simulink model "Lateral_control_of_HST"  (R2023b)
settings: Solver=ode45  StartTime=0.0  StopTime=100  FixedStep=0.001  RelTol=1e-3
InitFcn:
  | Parameters_and_initial_conditions;
values from neighbouring files (symbols this model uses):
  A_a = 2.119e-7    (= 2.119e-07)    [Parameters_and_initial_conditions.m]
  A_v = 4.032e-7    (= 4.032e-07)    [Parameters_and_initial_conditions.m]
  b = 0.7465    [Parameters_and_initial_conditions.m]
  c_px = 0    [Parameters_and_initial_conditions.m]
  c_py = 0    [Parameters_and_initial_conditions.m]
  c_pz = 1.5e4    (= 15000)    [Parameters_and_initial_conditions.m]
  c_sx = 0    [Parameters_and_initial_conditions.m]
  c_sy = 2e4    (= 20000)    [Parameters_and_initial_conditions.m]
  c_sz = 8e4    (= 80000)    [Parameters_and_initial_conditions.m]
  d_p = 1    [Parameters_and_initial_conditions.m]
  d_s = 1    [Parameters_and_initial_conditions.m]
  f_11 = 1.12e7    (= 11200000)    [Parameters_and_initial_conditions.m]
  f_22 = 9.98e6    (= 9980000)    [Parameters_and_initial_conditions.m]
  h_cs = 0.98    [Parameters_and_initial_conditions.m]
  h_ts = 0.0945    [Parameters_and_initial_conditions.m]
  h_tw = 0.1745    [Parameters_and_initial_conditions.m]
  J_cx = 89396    [Parameters_and_initial_conditions.m]
  J_cz = 2485756    [Parameters_and_initial_conditions.m]
  J_tx = 2650    [Parameters_and_initial_conditions.m]
  J_tz = 3000    [Parameters_and_initial_conditions.m]
  J_wz = 1200    [Parameters_and_initial_conditions.m]
  k11 = 1.88e7    (= 18800000)    [Parameters_and_initial_conditions.m]
  k12 = 5.807e5    (= 580700)    [Parameters_and_initial_conditions.m]
  k13 = 3.68e6    (= 3680000)    [Parameters_and_initial_conditions.m]
  k14 = 2.64e1    (= 26.4)    [Parameters_and_initial_conditions.m]
  k21 = 1.88e7    (= 18800000)    [Parameters_and_initial_conditions.m]
  k22 = 5.807e5    (= 580700)    [Parameters_and_initial_conditions.m]
  k23 = 3.68e6    (= 3680000)    [Parameters_and_initial_conditions.m]
  k24 = 2.64e1    (= 26.4)    [Parameters_and_initial_conditions.m]
  K_gpsi = -7834    [Parameters_and_initial_conditions.m]
  K_gy = 5014    [Parameters_and_initial_conditions.m]
  k_px = 1.45e7    (= 14500000)    [Parameters_and_initial_conditions.m]
  k_py = 7.5e6    (= 7500000)    [Parameters_and_initial_conditions.m]
  k_pz = 6.65e5    (= 665000)    [Parameters_and_initial_conditions.m]
  k_sx = 2.08e5    (= 208000)    [Parameters_and_initial_conditions.m]
  k_sy = 2.08e5    (= 208000)    [Parameters_and_initial_conditions.m]
  k_sz = 3.5e5    (= 350000)    [Parameters_and_initial_conditions.m]
  kd = 1    [Parameters_and_initial_conditions.m]
  kp = 3    [Parameters_and_initial_conditions.m]
  l = 9    [Parameters_and_initial_conditions.m]
  l_t = 1.25    [Parameters_and_initial_conditions.m]
  Lambda_a = 6.125e-7    (= 6.125e-07)    [Parameters_and_initial_conditions.m]
  lambda_e = 0.05    [Parameters_and_initial_conditions.m]
  Lambda_v = 1.08e-6    (= 1.08e-06)    [Parameters_and_initial_conditions.m]
  m_c = 40000    [Parameters_and_initial_conditions.m]
  m_t = 2280    [Parameters_and_initial_conditions.m]
  m_w = 1650    [Parameters_and_initial_conditions.m]
  Omega_c = 0.8246    [Parameters_and_initial_conditions.m]
  Omega_r = 0.0206    [Parameters_and_initial_conditions.m]
  Omega_s = 0.438    [Parameters_and_initial_conditions.m]
  psi_c_dot_initial = 0    [Parameters_and_initial_conditions.m]
  psi_c_initial = 0    [Parameters_and_initial_conditions.m]
  psi_t1_dot_initial = 0    [Parameters_and_initial_conditions.m]
  psi_t1_initial = 0    [Parameters_and_initial_conditions.m]
  psi_t2_dot_initial = 0    [Parameters_and_initial_conditions.m]
  psi_t2_initial = 0    [Parameters_and_initial_conditions.m]
  psi_w1_dot_initial = 0    [Parameters_and_initial_conditions.m]
  psi_w1_initial = 0    [Parameters_and_initial_conditions.m]
  psi_w2_dot_initial = 0    [Parameters_and_initial_conditions.m]
  psi_w2_initial = 0    [Parameters_and_initial_conditions.m]
  psi_w3_dot_initial = 0    [Parameters_and_initial_conditions.m]
  psi_w3_initial = 0    [Parameters_and_initial_conditions.m]
  psi_w4_dot_initial = 0    [Parameters_and_initial_conditions.m]
  psi_w4_initial = 0    [Parameters_and_initial_conditions.m]
  r_0 = 0.4575    [Parameters_and_initial_conditions.m]
  sigma = 0.05    [Parameters_and_initial_conditions.m]
  T1 = 0.15    [Parameters_and_initial_conditions.m]
  T2 = 0.04    [Parameters_and_initial_conditions.m]
  Tff = 0.1*tau    (= 0.3)    [Parameters_and_initial_conditions.m]
  Tff2 = 0.2*tau    (= 0.6)    [Parameters_and_initial_conditions.m]
  theta_c_dot_initial = 0    [Parameters_and_initial_conditions.m]
  theta_c_initial = 0    [Parameters_and_initial_conditions.m]
  theta_t1_dot_initial = 0    [Parameters_and_initial_conditions.m]
  theta_t1_initial = 0    [Parameters_and_initial_conditions.m]
  theta_t2_dot_initial = 0    [Parameters_and_initial_conditions.m]
  theta_t2_initial = 0    [Parameters_and_initial_conditions.m]
  Tnn = 0.5*tau    (= 1.5)    [Parameters_and_initial_conditions.m]
  Tnn2 = 1*tau    (= 3)    [Parameters_and_initial_conditions.m]
  V = 75    [Parameters_and_initial_conditions.m]
  y_c_dot_initial = 0    [Parameters_and_initial_conditions.m]
  y_c_initial = 0    [Parameters_and_initial_conditions.m]
  y_t1_dot_initial = 0    [Parameters_and_initial_conditions.m]
  y_t1_initial = 0    [Parameters_and_initial_conditions.m]
  y_t2_dot_initial = 0    [Parameters_and_initial_conditions.m]
  y_t2_initial = 0    [Parameters_and_initial_conditions.m]
  y_w1_dot_initial = 0    [Parameters_and_initial_conditions.m]
  y_w1_initial = 0    [Parameters_and_initial_conditions.m]
  y_w2_dot_initial = 0    [Parameters_and_initial_conditions.m]
  y_w2_initial = 0    [Parameters_and_initial_conditions.m]
  y_w3_dot_initial = 0    [Parameters_and_initial_conditions.m]
  y_w3_initial = 0    [Parameters_and_initial_conditions.m]
  y_w4_dot_initial = 0    [Parameters_and_initial_conditions.m]
  y_w4_initial = 0    [Parameters_and_initial_conditions.m]
libraries: simulink x6, dspsrcs4 x1
(part 1 of 2)
settings Model: Creator=Sky  LastModifiedBy=19534
settings SolverCC: AlgebraicLoopSolver=TrustRegion
settings DataIOCC: ReturnWorkspaceOutputs=off
settings DebuggingCC: UnconnectedInputMsg=warning  UnconnectedOutputMsg=warning  UnconnectedLineMsg=warning  ArithmeticOperatorsInVariantConditions=warning
settings ModelReferenceCC: EnableRefExpFcnMdlSchedulingChecks=on
settings SFSimCC: CustomCodeUndefinedFunction=UseInterfaceOnly

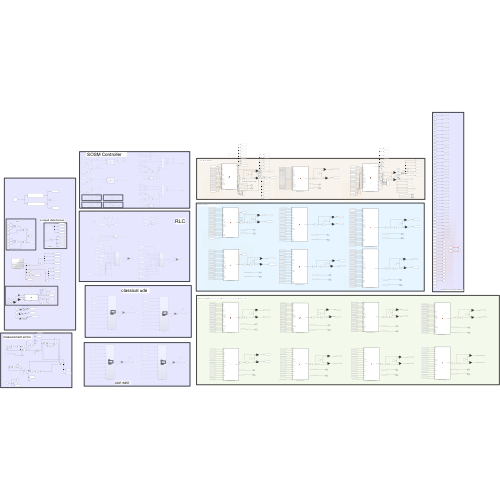
[thumbnail: Simulink's stored preview of the top-level diagram]
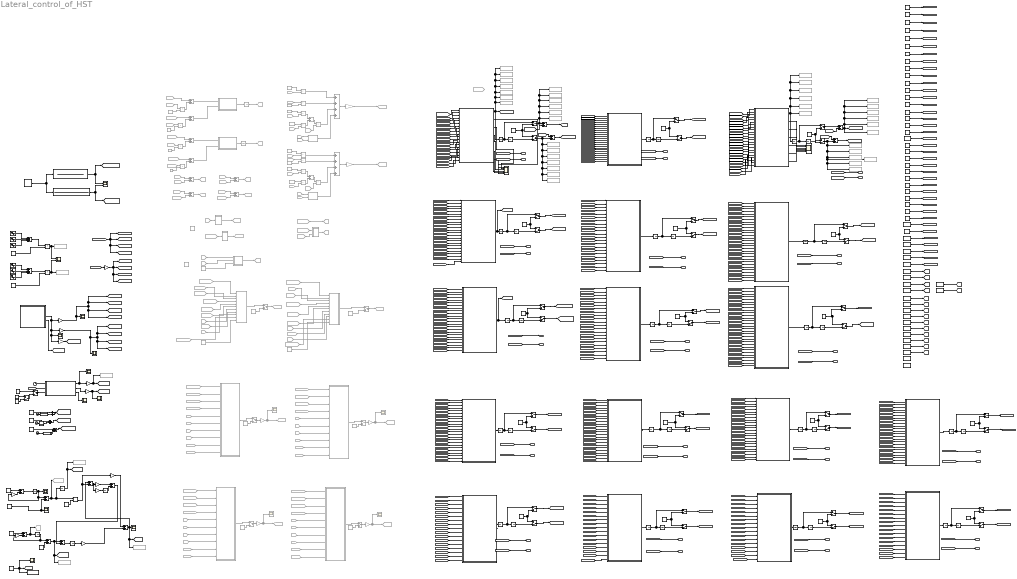
== system Lateral_control_of_HST ==
  note: classical ude
  note: 周期
  note: 非周期
  note: RLC
  note: 积分器的初值由外部m文件配置
  note: Car Body Dynamics
  note: Bogie Dynamics ( i = 1 , 2 )
  note: Wheelset Dynamics ( i = 1 , 2 , while j = 1 ; i = 3 , 4 , while j = 2 ) :
  note: Lumped disturbances
  note: measurement errors
  note: 这边是外部m文件中的系统参数导入simulink环境
  note: SOSM Controller
  note: X
  note: X_dot
  note: X_dot
  note: X
  note: UDE+MEE
  " " : Constant  Value=Lambda_v
  (3) : Sin  Amplitude=1/3  Frequency=2*pi  Phase=pi/2  SampleTime=0
  (35) : Sin  Amplitude=1/35  Frequency=6*pi  Phase=pi/2  SampleTime=0
  {0..1,23..26} (6 alike) : Constant  Commented=on  Value=0
  15 : Sin  Amplitude=1/15  Frequency=4*pi  Phase=pi/2  SampleTime=0
  3 : Sin  Amplitude=1/3  Frequency=2*pi  Phase=pi/2  SampleTime=0
  35 : Sin  Amplitude=1/35  Frequency=6*pi  Phase=pi/2  SampleTime=0
  4A_ap/pi : Constant  Value=4*0.01/pi
  4A_vp/b*pi : Constant  Value=4*0.01/(pi*0.7465)
  99 : Sin  Amplitude=1/99  Frequency=10*pi  Phase=pi/2  SampleTime=0
  Add : Sum  Inputs=+-+
  Add1 : Sum  Inputs=+++
  Add{9..10,14..21,24..25,49} (13 alike) : Sum
  Add{8,38..40,44,48} (6 alike) : Sum  Commented=on
  Add{41..42,45..46} (4 alike) : Sum  Commented=on  Inputs=+-
  Add43 : Sum  Commented=on  Inputs=++++
  Add47 : Sum  Commented=on  Inputs=++++
  Atan2 : Trigonometry  Operator=atan2
  Band-Limited White Noise : simulink/Sources/Band-Limited White Noise  Cov=[0.1]  Ts=0.001  seed=[100]
  Band-Limited White Noise1 : simulink/Sources/Band-Limited White Noise  Cov=[1e-12]  Ts=0.001  seed=[1001]
  Band-Limited White Noise4 : simulink/Sources/Band-Limited White Noise  Cov=[0.000000000418]  Ts=0.01  seed=[23341]
  Band-Limited White Noise5 : simulink/Sources/Band-Limited White Noise  Cov=[0.00000045]  Ts=0.01  seed=[23341]
  Band-Limited White Noise6 : simulink/Sources/Band-Limited White Noise  Cov=[0.00000000006985]  Ts=0.01  seed=[23341]
  Band-Limited White Noise7 : simulink/Sources/Band-Limited White Noise  Cov=[0.00000000487]  Ts=0.01  seed=[23341]
  Clock{2,9..10,17} (4 alike) : Clock
  Constant{1..17} (17 alike) : Constant  Value=0
  Constant19 : Constant  Commented=on  Value=0.25
  Constant21 : Constant  Commented=on  Value=0.25
  Constant{23,40,44..45,56..57} (6 alike) : Constant  Commented=on  Value=50
  Constant30 : Constant  Value=T1
  Constant33 : Constant  Value=T2
  Constant34 : Constant  Value=9.8
  Constant41 : Constant  Commented=on  Value=15
  Constant42 : Constant  Value=A_a
  Constant43 : Constant  Value=A_v
  Differential equation of psi_c : MATLAB Function  TreatAsAtomicUnit=on
  Differential equation of psi_t1 : MATLAB Function  TreatAsAtomicUnit=on
  Differential equation of psi_t2 : MATLAB Function  TreatAsAtomicUnit=on
  "Differential equation of psi_w1 " : MATLAB Function  TreatAsAtomicUnit=on
  Differential equation of psi_w2 : MATLAB Function  TreatAsAtomicUnit=on
  Differential equation of psi_w3 : MATLAB Function  TreatAsAtomicUnit=on
  Differential equation of psi_w4 : MATLAB Function  TreatAsAtomicUnit=on
  Differential equation of theta_c : MATLAB Function  TreatAsAtomicUnit=on
  Differential equation of theta_t1 : MATLAB Function  TreatAsAtomicUnit=on
  Differential equation of theta_t2 : MATLAB Function  TreatAsAtomicUnit=on
  Differential equation of y_c : MATLAB Function  TreatAsAtomicUnit=on
  Differential equation of y_t1 : MATLAB Function  TreatAsAtomicUnit=on
  Differential equation of y_t2 : MATLAB Function  TreatAsAtomicUnit=on
  Differential equation of y_w1 : MATLAB Function  TreatAsAtomicUnit=on
  Differential equation of y_w2 : MATLAB Function  TreatAsAtomicUnit=on
  Differential equation of y_w3 : MATLAB Function  TreatAsAtomicUnit=on
  Differential equation of y_w4 : MATLAB Function  TreatAsAtomicUnit=on
  F_wind : MATLAB Function  TreatAsAtomicUnit=on
  From1069 : From  Commented=on  GotoTag=noise_ddx
  From415 : From  Commented=on  GotoTag=K_sy
  From416 : From  Commented=on  GotoTag=C_sy
  From417 : From  Commented=on  GotoTag=M_c
  From418 : From  Commented=on  GotoTag=K_sy
  From419 : From  Commented=on  GotoTag=C_sy
  From420 : From  Commented=on  GotoTag=M_c
  From{423,812,817,822} (4 alike) : From  Commented=on  GotoTag=y_t1_dot
  From425 : From  Commented=on  GotoTag=y_t1
  From{426,428,435,803,819,829,854,861,881,884} (10 alike) : From  Commented=on  GotoTag=y_c
  From{427,430,436..437,813,815,821,831,855,863,882,886} (12 alike) : From  Commented=on  GotoTag=y_c_dot
  From429 : From  Commented=on  GotoTag=d_hat
  From431 : From  Commented=on  GotoTag=y_t2_dot
  From432 : From  Commented=on  GotoTag=y_t2
  From449 : From  Commented=on  GotoTag=d_hat
  From455 : From  Commented=on  GotoTag=z_1
  From457 : From  Commented=on  GotoTag=alpha_1_dot
  From466 : From  Commented=on  GotoTag=z_1
  From472 : From  Commented=on  GotoTag=alpha_1
  From474 : From  Commented=on  GotoTag=d_hat
  From475 : From  Commented=on  GotoTag=alpha_1_dot
  From476 : From  Commented=on  GotoTag=z_1
  From480 : From  Commented=on  GotoTag=z_2
  From804 : From  Commented=on  GotoTag=y_t1
  From814 : From  Commented=on  GotoTag=y_c_ddot
  From816 : From  Commented=on  GotoTag=y_t1_ddot
  From{818,828,833,839} (4 alike) : From  Commented=on  GotoTag=ic
  From820 : From  Commented=on  GotoTag=y_t1
  From823 : From  Commented=on  GotoTag=Xc1_dot
  From824 : From  Commented=on  GotoTag=Xc1
  From825 : From  Commented=on  GotoTag=Xc1_dot
  From826 : From  Commented=on  GotoTag=Xc1
  From827 : From  Commented=on  GotoTag=Xc1
  From830 : From  Commented=on  GotoTag=y_t2
  From832 : From  Commented=on  GotoTag=y_t2_dot
  From834 : From  Commented=on  GotoTag=Xc2_dot
  From835 : From  Commented=on  GotoTag=Xc2
  From836 : From  Commented=on  GotoTag=Xc2_dot
  From837 : From  Commented=on  GotoTag=Xc2
  From838 : From  Commented=on  GotoTag=Xc2
  From{856,869,883,890} (4 alike) : From  Commented=on  GotoTag=theta_c
  From{862,870,885,891} (4 alike) : From  Commented=on  GotoTag=theta_c_dot
  From864 : From  Commented=on  GotoTag=k21
  From865 : From  Commented=on  GotoTag=k22
  From868 : From  Commented=on  GotoTag=k23
  From871 : From  Commented=on  GotoTag=k24
  From{872,878,893,899} (4 alike) : From  Commented=on  GotoTag=f_1
  From{873,879,894,900} (4 alike) : From  Commented=on  GotoTag=f_2
  From874 : From  Commented=on  GotoTag=k11
  From875 : From  Commented=on  GotoTag=k12
  From876 : From  Commented=on  GotoTag=k13
  From877 : From  Commented=on  GotoTag=k14
  From887 : From  Commented=on  GotoTag=k11
  From888 : From  Commented=on  GotoTag=k12
  From889 : From  Commented=on  GotoTag=k13
  From892 : From  Commented=on  GotoTag=k14
  From895 : From  Commented=on  GotoTag=k11
  From896 : From  Commented=on  GotoTag=k12
  From897 : From  Commented=on  GotoTag=k13
  From898 : From  Commented=on  GotoTag=k14
  Gain{,3..4,6,10,21} (6 alike) : Gain
  Gain1 : Gain  Gain=5
  Gain2 : Gain  Gain=0.04
  Gain23 : Gain  Commented=on  Gain=16.7
  Gain24 : Gain  Commented=on  Gain=16.7
  Gain{26..29} (4 alike) : Gain  Commented=on
  Gain5 : Gain  Gain=0
  Gain7 : Gain  Gain=-0.01315789
  Gain8 : Gain  Gain=-0.05263158
  Gain9 : Gain  Gain=0.001
  Goto154 : Goto  Commented=on  GotoTag=noise_ddx
  Goto155 : Goto  Commented=on  GotoTag=noise_ddphi
  Goto162 : Goto  Commented=on  GotoTag=ic
  Goto163 : Goto  Commented=on  GotoTag=it
  Goto164 : Goto  Commented=on  GotoTag=Xc1
  Goto165 : Goto  Commented=on  GotoTag=Xc1_dot
  Goto{45,166,176,181} (4 alike) : Goto  Commented=on  GotoTag=f_1
  Goto167 : Goto  Commented=on  GotoTag=Xc2
  Goto168 : Goto  Commented=on  GotoTag=Xc2_dot
  Goto17 : Goto  Commented=on  GotoTag=z_1
  Goto{48,173,179,182} (4 alike) : Goto  Commented=on  GotoTag=f_2
  Goto20 : Goto  Commented=on  GotoTag=d_hat
  Goto39 : Goto  Commented=on  GotoTag=alpha_1
  Goto42 : Goto  Commented=on  GotoTag=alpha_1_dot
  Goto51 : Goto  Commented=on  GotoTag=z_2
  Integrator : Integrator  InitialCondition=y_c_dot_initial
  Integrator1 : Integrator  InitialCondition=y_c_initial
  Integrator10 : Integrator  InitialCondition=psi_t1_dot_initial
  Integrator11 : Integrator  InitialCondition=psi_t1_initial
  Integrator12 : Integrator  InitialCondition=psi_t2_initial
  Integrator13 : Integrator  InitialCondition=psi_t2_dot_initial
  Integrator14 : Integrator  InitialCondition=theta_t1_dot_initial
  Integrator15 : Integrator  InitialCondition=theta_t1_initial
  Integrator16 : Integrator  InitialCondition=theta_t2_dot_initial
  Integrator17 : Integrator  InitialCondition=theta_t2_initial
  Integrator18 : Integrator  InitialCondition=y_w1_dot_initial
  Integrator19 : Integrator  InitialCondition=y_w1_initial
  Integrator2 : Integrator  InitialCondition=psi_c_dot_initial
  Integrator20 : Integrator  InitialCondition=y_w2_dot_initial
  Integrator21 : Integrator  InitialCondition=y_w2_initial
  Integrator22 : Integrator  InitialCondition=y_w3_dot_initial
  Integrator23 : Integrator  InitialCondition=y_w3_initial
  Integrator24 : Integrator  InitialCondition=y_w4_initial
  Integrator25 : Integrator  InitialCondition=y_w4_dot_initial
  Integrator26 : Integrator  InitialCondition=psi_w1_dot_initial
  Integrator27 : Integrator  InitialCondition=psi_w1_initial
  Integrator28 : Integrator  InitialCondition=psi_w2_dot_initial
  Integrator29 : Integrator  InitialCondition=psi_w2_initial
  Integrator3 : Integrator  InitialCondition=psi_c_initial
  Integrator30 : Integrator  InitialCondition=psi_w3_dot_initial
  Integrator31 : Integrator  InitialCondition=psi_w3_initial
  Integrator32 : Integrator  InitialCondition=psi_w4_dot_initial
  Integrator33 : Integrator  InitialCondition=psi_w4_initial
  Integrator{34..38} (5 alike) : Integrator
  Integrator4 : Integrator  InitialCondition=theta_c_dot_initial
  Integrator41 : Integrator  Commented=on  LimitOutput=on  UpperSaturationLimit=80  LowerSaturationLimit=0
  Integrator42 : Integrator  Commented=on
  Integrator5 : Integrator  InitialCondition=theta_c_initial
  Integrator6 : Integrator  InitialCondition=y_t1_dot_initial
  Integrator7 : Integrator  InitialCondition=y_t1_initial
  Integrator8 : Integrator  InitialCondition=y_t2_dot_initial
  Integrator9 : Integrator  InitialCondition=y_t2_initial
  J_cx : Constant  Value=J_cx
  J_cz : Constant  Value=J_cz
  "J_tx " : Constant  Value=J_tx
  "J_tz " : Constant  Value=J_tz
  J_wz : Constant  Value=J_wz
  K_gpsi : Constant  Value=K_gpsi
  K_gy : Constant  Value=K_gy
  Lambda_a : Constant  Value=Lambda_a
  MATLAB Function10 : MATLAB Function  Commented=on  TreatAsAtomicUnit=on
  MATLAB Function16 : MATLAB Function  TreatAsAtomicUnit=on
  MATLAB Function5 : MATLAB Function  Commented=on  TreatAsAtomicUnit=on
  MATLAB Function6 : MATLAB Function  Commented=on  TreatAsAtomicUnit=on
  MATLAB Function7 : MATLAB Function  Commented=on  TreatAsAtomicUnit=on
  MATLAB Function8 : MATLAB Function  TreatAsAtomicUnit=on
  MATLAB Function9 : MATLAB Function  TreatAsAtomicUnit=on
  M_t : Constant  Value=m_t
  M_w : Constant  Value=m_w
  Manual Switch{,35,56..59} (6 alike) : ManualSwitch  Commented=on
  Manual Switch{1..2,4,6,8,10,12,14,16,18,20,22,24,26,28,30,32,54} (18 alike) : ManualSwitch
  Manual Switch{3,5,7,9,11,13,15,17,19,21,23,25,27,29,31,33..34,53} (18 alike) : ManualSwitch  CurrentSetting=0
  Omega_c : Constant  Value=Omega_c
  Omega_r : Constant  Value=Omega_r
  Omega_s : Constant  Value=Omega_s
  Product1 : Product
  Product24 : Product
  Product{46..59} (14 alike) : Product  Commented=on
  Scope : Scope  NumInputPorts=2
  Scope1 : Scope  NumInputPorts=2
  Scope{10,14,33..34} (4 alike) : Scope  Commented=on
  Scope{2..4,7..8,25,30..32,35} (10 alike) : Scope
  Scope40 : Scope  NumInputPorts=6
  Scope49 : Scope  NumInputPorts=6
  Subsystem10 : Subsystem  Commented=on
  Subsystem11 : Subsystem  Commented=on
  Subsystem3 : Subsystem  Commented=on
  Subsystem7 : Subsystem  Commented=on
  Subsystem8 : Subsystem  Commented=on
  Subsystem9 : Subsystem  Commented=on
  Subtract : Sum  Inputs=+-
  Subtract1 : Sum  Inputs=+-
  Tff : Constant  Value=Tff
  Tff2 : Constant  Value=Tff2
  Tnn : Constant  Value=Tnn
  Tnn2 : Constant  Value=Tnn2
  To Workspace1 : ToWorkspace  Commented=on  VariableName=wind_20  SaveFormat=Timeseries  SampleTime=-1
  To Workspace10 : ToWorkspace  Commented=on  VariableName=v_passive_n  SaveFormat=Timeseries  SampleTime=-1
  To Workspace11 : ToWorkspace  Commented=on  VariableName=acc_passive_n  SaveFormat=Timeseries  SampleTime=-1
  To Workspace12 : ToWorkspace  Commented=on  VariableName=acc_sosm_n  SaveFormat=Timeseries  SampleTime=-1
  To Workspace13 : ToWorkspace  Commented=on  VariableName=acc_rlc_n  SaveFormat=Timeseries  SampleTime=-1
  To Workspace14 : ToWorkspace  Commented=on  VariableName=acc_ude_n  SaveFormat=Timeseries  SampleTime=-1
  To Workspace15 : ToWorkspace  Commented=on  VariableName=pacc_sosm_n  SaveFormat=Timeseries  SampleTime=-1
  To Workspace16 : ToWorkspace  Commented=on  VariableName=acc_mee  SaveFormat=Timeseries  SampleTime=-1
  To Workspace17 : ToWorkspace  Commented=on  VariableName=v_sosm_n  SaveFormat=Timeseries  SampleTime=-1
  To Workspace18 : ToWorkspace  Commented=on  VariableName=theta_cl  SaveFormat=Timeseries  SampleTime=-1
  To Workspace19 : ToWorkspace  Commented=on  VariableName=noise_v  SaveFormat=Timeseries  SampleTime=-1
  To Workspace2 : ToWorkspace  Commented=on  VariableName=phic_v_sosm_n  SaveFormat=Timeseries  SampleTime=-1
  To Workspace20 : ToWorkspace  Commented=on  VariableName=noise_w  SaveFormat=Timeseries  SampleTime=-1
  To Workspace21 : ToWorkspace  Commented=on  VariableName=v_rlc_n  SaveFormat=Timeseries  SampleTime=-1
  To Workspace22 : ToWorkspace  Commented=on  VariableName=v_ude_n  SaveFormat=Timeseries  SampleTime=-1
  To Workspace23 : ToWorkspace  Commented=on  VariableName=v_mee  SaveFormat=Timeseries  SampleTime=-1
  To Workspace24 : ToWorkspace  Commented=on  VariableName=phic_sosm_n  SaveFormat=Timeseries  SampleTime=-1
  To Workspace25 : ToWorkspace  Commented=on  VariableName=phic_rlc_n  SaveFormat=Timeseries  SampleTime=-1
  To Workspace26 : ToWorkspace  Commented=on  VariableName=phic_ude_n  SaveFormat=Timeseries  SampleTime=-1
  To Workspace27 : ToWorkspace  Commented=on  VariableName=phic_mee  SaveFormat=Timeseries  SampleTime=-1
  To Workspace28 : ToWorkspace  Commented=on  VariableName=phic_v_rlc_n  SaveFormat=Timeseries  SampleTime=-1
  To Workspace29 : ToWorkspace  Commented=on  VariableName=phic_v_ude_n  SaveFormat=Timeseries  SampleTime=-1
  To Workspace3 : ToWorkspace  Commented=on  VariableName=ya  SaveFormat=Timeseries  SampleTime=-1
  To Workspace30 : ToWorkspace  Commented=on  VariableName=phic_v_mee  SaveFormat=Timeseries  SampleTime=-1
  To Workspace31 : ToWorkspace  Commented=on  VariableName=phic_v_passive_n  SaveFormat=Timeseries  SampleTime=-1
  To Workspace32 : ToWorkspace  Commented=on  VariableName=pacc_rlc_n  SaveFormat=Timeseries  SampleTime=-1
  To Workspace33 : ToWorkspace  Commented=on  VariableName=pacc_ude_n  SaveFormat=Timeseries  SampleTime=-1
  To Workspace34 : ToWorkspace  Commented=on  VariableName=pacc_mee  SaveFormat=Timeseries  SampleTime=-1
  To Workspace35 : ToWorkspace  Commented=on  VariableName=pacc_passive_n  SaveFormat=Timeseries  SampleTime=-1
  To Workspace36 : ToWorkspace  Commented=on  VariableName=acc_tau_5  SaveFormat=Timeseries  SampleTime=-1
  To Workspace37 : ToWorkspace  Commented=on  VariableName=yc_tau_10  SaveFormat=Timeseries  SampleTime=-1
  To Workspace38 : ToWorkspace  Commented=on  VariableName=acc_mee_n  SaveFormat=Timeseries  SampleTime=-1
  To Workspace39 : ToWorkspace  Commented=on  VariableName=yc_mee_n  SaveFormat=Timeseries  SampleTime=-1
  To Workspace4 : ToWorkspace  Commented=on  VariableName=yc_passive_n  SaveFormat=Timeseries  SampleTime=-1
  To Workspace40 : ToWorkspace  Commented=on  VariableName=pacc_mee_n  SaveFormat=Timeseries  SampleTime=-1
  To Workspace41 : ToWorkspace  Commented=on  VariableName=phic_mee_n  SaveFormat=Timeseries  SampleTime=-1
  To Workspace42 : ToWorkspace  Commented=on  VariableName=phic_v_mee_n  SaveFormat=Timeseries  SampleTime=-1
  To Workspace43 : ToWorkspace  Commented=on  VariableName=v_mee_n  SaveFormat=Timeseries  SampleTime=-1
  To Workspace44 : ToWorkspace  Commented=on  VariableName=noise_theata  SaveFormat=Timeseries  SampleTime=-1
  To Workspace46 : ToWorkspace  VariableName=yczaosheng  SaveFormat=Timeseries  SampleTime=-1
  To Workspace5 : ToWorkspace  Commented=on  VariableName=phic_passive_n  SaveFormat=Timeseries  SampleTime=-1
  To Workspace6 : ToWorkspace  Commented=on  VariableName=yc_sosm_n  SaveFormat=Timeseries  SampleTime=-1
  To Workspace7 : ToWorkspace  Commented=on  VariableName=yc_rlc_n  SaveFormat=Timeseries  SampleTime=-1
  To Workspace8 : ToWorkspace  Commented=on  VariableName=yc_ude_n  SaveFormat=Timeseries  SampleTime=-1
  To Workspace9 : ToWorkspace  Commented=on  VariableName=yc_mee  SaveFormat=Timeseries  SampleTime=-1
  Transfer Fcn2 : TransferFcn  Numerator=[sqrt(2*pi*A_a*V^3*Omega_c^2)]  Denominator=conv([1 V*Omega_r], [1 V*Omega_c])
  Transfer Fcn3 : TransferFcn  Numerator=[sqrt(2*pi*A_v*b^-2*V^3*Omega_c^2) 0]  Denominator=conv(conv([1 V*Omega_r], [1 V*Omega_c]), [1 V*Omega_s])
  UDE+MEE4（新）10 : Subsystem  Commented=on
  UDE+MEE4（新）8 : Subsystem  Commented=on
  UDE1 : Subsystem  Commented=on
  UDE2 : Subsystem  Commented=on
  V : Constant  Value=V
  b : Constant  Value=b
  c4 : Constant  Commented=on  Value=1232*6
  c5 : Constant  Commented=on  Value=1929*6
  c6 : Constant  Commented=on  Value=1232*6
  c7 : Constant  Commented=on  Value=1929*6
  c_px : Constant  Value=c_px
  c_py : Constant  Value=c_py
  "c_pz " : Constant  Value=c_pz
  c_sx : Constant  Value=c_sx
  "c_sy " : Constant  Value=c_sy
  "c_sz " : Constant  Value=c_sz
  d_p : Constant  Value=d_p
  d_s : Constant  Value=d_s
  disturbance and noise : Subsystem
  f_11 : Constant  Value=f_11
  f_22 : Constant  Value=f_22
  h_cs : Constant  Value=h_cs
  "h_ts " : Constant  Value=h_ts
  h_tw : Constant  Value=h_tw
  k1 : Constant  Value=k21
  k1'2 : Constant  Commented=on  Value=1929*6
  k1'3 : Constant  Commented=on  Value=1929*6
  k11 : Constant  Value=k11
  k12 : Constant  Value=k12
  k13 : Constant  Value=k13
  k14 : Constant  Value=k14
  k2 : Constant  Value=k22
  k23 : Constant  Value=k23
  k24 : Constant  Value=k24
  k4 : Constant  Commented=on  Value=5100*6
  k5 : Constant  Commented=on  Value=5100*6
  k_px : Constant  Value=k_px
  "k_py " : Constant  Value=k_py
  k_pz : Constant  Value=k_pz
  k_sx : Constant  Value=k_sx
  k_sy : Constant  Value=k_sy
  k_sz : Constant  Value=k_sz
  kd : Constant  Value=kd
  kp : Constant  Value=kp
  l_c : Constant  Value=l
  l_t : Constant  Value=l_t
  lambda_e : Constant  Value=lambda_e
  m_c : Constant  Value=m_c
  r_0 : Constant  Value=r_0
  sigma : Constant  Value=sigma
  w_wind : Constant  Value=0
  w_wind1 : Constant  Value=10
  w_wind4 : Constant  Value=20
  y_c : Outport  VectorParamsAs1DForOutWhenUnconnected=off
  y_c_dot : Outport  Port=2  VectorParamsAs1DForOutWhenUnconnected=off
  psi_c : Outport  Port=3  VectorParamsAs1DForOutWhenUnconnected=off
  psi_c_dot : Outport  Port=4  VectorParamsAs1DForOutWhenUnconnected=off
  theta_c : Outport  Port=5  VectorParamsAs1DForOutWhenUnconnected=off
  theta_c_dot : Outport  Port=6  VectorParamsAs1DForOutWhenUnconnected=off
  y_t1 : Outport  Port=7  VectorParamsAs1DForOutWhenUnconnected=off
  y_t1_dot : Outport  Port=8  VectorParamsAs1DForOutWhenUnconnected=off
  y_t2 : Outport  Port=9  VectorParamsAs1DForOutWhenUnconnected=off
  y_t2_dot : Outport  Port=10  VectorParamsAs1DForOutWhenUnconnected=off
  psi_t1 : Outport  Port=11  VectorParamsAs1DForOutWhenUnconnected=off
  psi_t1_dot : Outport  Port=12  VectorParamsAs1DForOutWhenUnconnected=off
  psi_t2 : Outport  Port=13  VectorParamsAs1DForOutWhenUnconnected=off
  psi_t2_dot : Outport  Port=14  VectorParamsAs1DForOutWhenUnconnected=off
  theta_t1 : Outport  Port=15  VectorParamsAs1DForOutWhenUnconnected=off
  theta_t1_dot : Outport  Port=16  VectorParamsAs1DForOutWhenUnconnected=off
  theta_t2 : Outport  Port=17  VectorParamsAs1DForOutWhenUnconnected=off
  theta_t2_dot : Outport  Port=18  VectorParamsAs1DForOutWhenUnconnected=off
  y_w1 : Outport  Port=19  VectorParamsAs1DForOutWhenUnconnected=off
  y_w1_dot : Outport  Port=20  VectorParamsAs1DForOutWhenUnconnected=off
  y_w2 : Outport  Port=21  VectorParamsAs1DForOutWhenUnconnected=off
  y_w2_dot : Outport  Port=22  VectorParamsAs1DForOutWhenUnconnected=off
  y_w3 : Outport  Port=23  VectorParamsAs1DForOutWhenUnconnected=off
  y_w3_dot : Outport  Port=24  VectorParamsAs1DForOutWhenUnconnected=off
  y_w4 : Outport  Port=25  VectorParamsAs1DForOutWhenUnconnected=off
  y_w4_dot : Outport  Port=26  VectorParamsAs1DForOutWhenUnconnected=off
  psi_w1 : Outport  Port=27  VectorParamsAs1DForOutWhenUnconnected=off
  psi_w1_dot : Outport  Port=28  VectorParamsAs1DForOutWhenUnconnected=off
  psi_w2 : Outport  Port=29  VectorParamsAs1DForOutWhenUnconnected=off
  psi_w2_dot : Outport  Port=30  VectorParamsAs1DForOutWhenUnconnected=off
  psi_w3 : Outport  Port=31  VectorParamsAs1DForOutWhenUnconnected=off
  psi_w3_dot : Outport  Port=32  VectorParamsAs1DForOutWhenUnconnected=off
  psi_w4 : Outport  Port=33  VectorParamsAs1DForOutWhenUnconnected=off
  psi_w4_dot : Outport  Port=34  VectorParamsAs1DForOutWhenUnconnected=off
  wires:
  [y_c] -> Differential equation of y_c/3(y_c)
  [f_1] -> Differential equation of y_c/18(f_1)
  [f_2] -> Differential equation of y_c/19(f_2)
  [psi_c] -> Differential equation of psi_c/3(psi_c)
  [psi_c_dot] -> Differential equation of psi_c/4(psi_c_dot)
  [f_1] -> Differential equation of psi_c/23(f_1)
  [f_2] -> Differential equation of psi_c/24(f_2)
  [psi_c] -> psi_c/1
  [psi_c_dot] -> psi_c_dot/1
  [y_c_dot] -> y_c_dot/1
  Integrator4/1 -> Manual Switch2/1, Integrator5/1  "d_phi_real"
  [theta_c] -> Differential equation of theta_c/5(theta_c)
  [theta_c_dot] -> Differential equation of theta_c/13(theta_c_dot)
  [y_c_dot] -> Differential equation of theta_c/12(y_c_dot)
  [theta_c_dot] -> Differential equation of y_c/13(theta_c_dot)
  [theta_c] -> Differential equation of y_c/5(theta_c)
  [y_c] -> Differential equation of theta_c/3(y_c)
  [theta_c] -> theta_c/1
  [theta_c_dot] -> theta_c_dot/1
  Differential equation of y_t1/1(y_t1_ddot) -> [y_t1_ddot], Integrator6/1
  [psi_c] -> Differential equation of y_t1/5(psi_c)
  Differential equation of y_t2/1(y_t2_ddot) -> [y_t2_ddot], Integrator8/1
  [y_t2] -> y_t2/1
  [y_t2_dot] -> y_t2_dot/1
  [y_t1_dot] -> y_t1_dot/1
  [y_t1] -> y_t1/1
  Differential equation of psi_t1/1(psi_t1_ddot) -> Integrator10/1
  [psi_t1_dot] -> psi_t1_dot/1
  [psi_t1] -> psi_t1/1
  Differential equation of psi_t2/1(psi_t2_ddot) -> Integrator13/1
  [psi_t2] -> psi_t2/1
  [psi_t2_dot] -> psi_t2_dot/1
  Differential equation of theta_t1/1(theta_t1_ddot) -> Integrator14/1
  [theta_t1] -> theta_t1/1
  [theta_t1_dot] -> theta_t1_dot/1
  Differential equation of theta_t2/1(theta_t2_ddot) -> Integrator16/1
  [theta_t2] -> theta_t2/1
  [theta_t2_dot] -> theta_t2_dot/1
  Differential equation of y_w1/1(y_w1_ddot) -> Integrator18/1
  [y_w1_dot] -> y_w1_dot/1
  [y_w1] -> y_w1/1
  Differential equation of y_w2/1(y_w2_ddot) -> Integrator20/1
  [y_w2_dot] -> y_w2_dot/1
  [y_w2] -> y_w2/1
  Differential equation of y_w3/1(y_w3_ddot) -> Integrator22/1
  [y_w3_dot] -> y_w3_dot/1
  [y_w3] -> y_w3/1
  Differential equation of y_w4/1(y_w4_ddot) -> Integrator25/1
  [y_w4_dot] -> y_w4_dot/1
  [y_w4] -> y_w4/1
  "Differential equation of psi_w1 "/1(psi_w1_ddot) -> Integrator26/1
  [psi_w1_dot] -> psi_w1_dot/1
  [psi_w1] -> psi_w1/1
  Differential equation of psi_w2/1(psi_w2_ddot) -> Integrator28/1
  [psi_w2_dot] -> psi_w2_dot/1
  [psi_w2] -> psi_w2/1
  Differential equation of psi_w3/1(psi_w3_ddot) -> Integrator30/1
  [psi_w3_dot] -> psi_w3_dot/1
  [psi_w3] -> psi_w3/1
  Differential equation of psi_w4/1(psi_w4_ddot) -> Integrator32/1
  [psi_w4_dot] -> psi_w4_dot/1
  [psi_w4] -> psi_w4/1
  [M_c] -> Differential equation of y_c/1(m_c)
  [h_cs] -> Differential equation of y_c/4(h_cs)
  [y_t1] -> Differential equation of y_c/6(y_t1)
  [y_t2] -> Differential equation of y_c/7(y_t2)
  [h_ts] -> Differential equation of y_c/8(h_ts)
  [theta_t1] -> Differential equation of y_c/9(theta_t1)
  [C_sy] -> Differential equation of y_c/11(c_sy)
  [theta_t2] -> Differential equation of y_c/10(theta_t2)
  [y_t1_dot] -> Differential equation of y_c/14(y_t1_dot)
  [y_t2_dot] -> Differential equation of y_c/15(y_t2_dot)
  [theta_t2_dot] -> Differential equation of y_c/17(theta_t2_dot)
  [theta_t1_dot] -> Differential equation of y_c/16(theta_t1_dot)
  [J_cz] -> Differential equation of psi_c/1(J_cz)
  [k_sx] -> Differential equation of psi_c/2(k_sx)
  [psi_t1] -> Differential equation of psi_c/5(psi_t1)
  [psi_t2] -> Differential equation of psi_c/6(psi_t2)
  [d_s] -> Differential equation of psi_c/7(d_s)
  [c_sx] -> Differential equation of psi_c/8(c_sx)
  [psi_t1_dot] -> Differential equation of psi_c/9(psi_t1_dot)
  [psi_t2_dot] -> Differential equation of psi_c/10(psi_t2_dot)
  [K_sy] -> Differential equation of psi_c/11(k_sy)
  [l] -> Differential equation of psi_c/12(l)
  [y_t1] -> Differential equation of psi_c/13(y_t1)
  [y_t1_dot] -> Differential equation of psi_c/14(y_t1_dot)
  [y_t2] -> Differential equation of psi_c/15(y_t2)
  [y_t2_dot] -> Differential equation of psi_c/16(y_t2_dot)
  [h_ts] -> Differential equation of psi_c/17(h_ts)
  [theta_t1] -> Differential equation of psi_c/18(theta_t1)
  [theta_t1_dot] -> Differential equation of psi_c/19(theta_t1_dot)
  [theta_t2] -> Differential equation of psi_c/20(theta_t2)
  [theta_t2_dot] -> Differential equation of psi_c/21(theta_t2_dot)
  [C_sy] -> Differential equation of psi_c/22(c_sy)
  [K_sy] -> Differential equation of y_c/2(k_sy)
  [m_w] -> Differential equation of y_w1/1(m_w)
  [k_py] -> Differential equation of y_w1/2(k_py)
  [y_t1] -> Differential equation of y_w1/3(y_t1)
  [b] -> Differential equation of y_w1/4(b)
  [psi_t1] -> Differential equation of y_w1/5(psi_t1)
  [h_tp] -> Differential equation of y_w1/6(h_tp)
  [theta_t1] -> Differential equation of y_w1/7(theta_t1)
  [y_w1] -> Differential equation of y_w1/8(y_w1)
  [c_py] -> Differential equation of y_w1/9(c_py)
  [y_t1_dot] -> Differential equation of y_w1/10(y_t1_dot)
  [psi_t1_dot] -> Differential equation of y_w1/11(psi_t1_dot)
  [theta_t1_dot] -> Differential equation of y_w1/12(theta_t1_dot)
  [y_w1_dot] -> Differential equation of y_w1/13(y_w1_dot)
  [f_22] -> Differential equation of y_w1/14(f_22)
  [V] -> Differential equation of y_w1/15(V)
  [sigma] -> Differential equation of y_w1/16(sigma)
  [r_0] -> Differential equation of y_w1/17(r_0)
  [a] -> Differential equation of y_w1/18(a)
  [y_a1_dot] -> Differential equation of y_w1/19(y_a1_dot)
  [theta_cl1_dot] -> Differential equation of y_w1/20(theta_cl1_dot)
  [psi_w1] -> Differential equation of y_w1/21(psi_w1)
  [K_gy] -> Differential equation of y_w1/22(K_gy)
  [y_a1] -> Differential equation of y_w1/23(y_a1)
  [theta_cl1] -> Differential equation of y_w1/24(theta_cl1)
  [J_wz] -> "Differential equation of psi_w1 "/1(J_wz)
  [k_px] -> "Differential equation of psi_w1 "/2(k_px)
  [psi_t1] -> "Differential equation of psi_w1 "/3(psi_t1)
  [psi_w1] -> "Differential equation of psi_w1 "/4(psi_w1)
  [d_p] -> "Differential equation of psi_w1 "/5(d_p)
  [c_px] -> "Differential equation of psi_w1 "/6(c_px)
  [psi_t1_dot] -> "Differential equation of psi_w1 "/7(psi_t1_dot)
  [psi_w1_dot] -> "Differential equation of psi_w1 "/8(psi_w1_dot)
  [f_11] -> "Differential equation of psi_w1 "/9(f_11)
  [lambda_e] -> "Differential equation of psi_w1 "/10(lambda_e)
  [y_w1] -> "Differential equation of psi_w1 "/11(y_w1)
  [y_a1] -> "Differential equation of psi_w1 "/12(y_a1)
  [theta_cl1] -> "Differential equation of psi_w1 "/13(theta_cl1)
  [V] -> "Differential equation of psi_w1 "/14(V)
  [K_gpsi] -> "Differential equation of psi_w1 "/15(K_gpsi)
  [J_wz] -> Differential equation of psi_w2/1(J_wz)
  [k_px] -> Differential equation of psi_w2/2(k_px)
  [psi_t1] -> Differential equation of psi_w2/3(psi_t1)
  [psi_w2] -> Differential equation of psi_w2/4(psi_w2)
  [d_p] -> Differential equation of psi_w2/5(d_p)
  [c_px] -> Differential equation of psi_w2/6(c_px)
  [psi_t1_dot] -> Differential equation of psi_w2/7(psi_t1_dot)
  [psi_w2_dot] -> Differential equation of psi_w2/8(psi_w2_dot)
  [f_11] -> Differential equation of psi_w2/9(f_11)
  [lambda_e] -> Differential equation of psi_w2/10(lambda_e)
  [y_w2] -> Differential equation of psi_w2/11(y_w2)
  [y_a2] -> Differential equation of psi_w2/12(y_a2)
  [theta_cl2] -> Differential equation of psi_w2/13(theta_cl2)
  [V] -> Differential equation of psi_w2/14(V)
  [K_gpsi] -> Differential equation of psi_w2/15(K_gpsi)
  [J_wz] -> Differential equation of psi_w3/1(J_wz)
  [psi_t2] -> Differential equation of psi_w3/3(psi_t2)
  [k_px] -> Differential equation of psi_w3/2(k_px)
  [d_p] -> Differential equation of psi_w3/5(d_p)
  [psi_w3] -> Differential equation of psi_w3/4(psi_w3)
  [c_px] -> Differential equation of psi_w3/6(c_px)
  [psi_t2_dot] -> Differential equation of psi_w3/7(psi_t2_dot)
  [psi_w3_dot] -> Differential equation of psi_w3/8(psi_w3_dot)
  [f_11] -> Differential equation of psi_w3/9(f_11)
  [lambda_e] -> Differential equation of psi_w3/10(lambda_e)
  [y_w3] -> Differential equation of psi_w3/11(y_w3)
  [y_a3] -> Differential equation of psi_w3/12(y_a3)
  [theta_cl3] -> Differential equation of psi_w3/13(theta_cl3)
  [V] -> Differential equation of psi_w3/14(V)
  [K_gpsi] -> Differential equation of psi_w3/15(K_gpsi)
  [J_wz] -> Differential equation of psi_w4/1(J_wz)
  [k_px] -> Differential equation of psi_w4/2(k_px)
  [psi_t2] -> Differential equation of psi_w4/3(psi_t2)
  [psi_w4] -> Differential equation of psi_w4/4(psi_w4)
  [d_p] -> Differential equation of psi_w4/5(d_p)
  [c_px] -> Differential equation of psi_w4/6(c_px)
  [psi_t2_dot] -> Differential equation of psi_w4/7(psi_t2_dot)
  [psi_w4_dot] -> Differential equation of psi_w4/8(psi_w4_dot)
  [f_11] -> Differential equation of psi_w4/9(f_11)
  [lambda_e] -> Differential equation of psi_w4/10(lambda_e)
  [y_w4] -> Differential equation of psi_w4/11(y_w4)
  [y_a4] -> Differential equation of psi_w4/12(y_a4)
  [theta_cl4] -> Differential equation of psi_w4/13(theta_cl4)
  [V] -> Differential equation of psi_w4/14(V)
  [K_gpsi] -> Differential equation of psi_w4/15(K_gpsi)
  [m_w] -> Differential equation of y_w2/1(m_w)
  [k_py] -> Differential equation of y_w2/2(k_py)
  [y_t1] -> Differential equation of y_w2/3(y_t1)
  [b] -> Differential equation of y_w2/4(b)
  [psi_t1] -> Differential equation of y_w2/5(psi_t1)
  [h_tp] -> Differential equation of y_w2/6(h_tp)
  [theta_t1] -> Differential equation of y_w2/7(theta_t1)
  [y_w2] -> Differential equation of y_w2/8(y_w2)
  [c_py] -> Differential equation of y_w2/9(c_py)
  [psi_t1_dot] -> Differential equation of y_w2/11(psi_t1_dot)
  [y_t1_dot] -> Differential equation of y_w2/10(y_t1_dot)
  [theta_t1_dot] -> Differential equation of y_w2/12(theta_t1_dot)
  [y_w2_dot] -> Differential equation of y_w2/13(y_w2_dot)
  [V] -> Differential equation of y_w2/15(V)
  [f_22] -> Differential equation of y_w2/14(f_22)
  [sigma] -> Differential equation of y_w2/16(sigma)
  [r_0] -> Differential equation of y_w2/17(r_0)
  [a] -> Differential equation of y_w2/18(a)
  [y_a2_dot] -> Differential equation of y_w2/19(y_a2_dot)
  [theta_cl2_dot] -> Differential equation of y_w2/20(theta_cl2_dot)
  [psi_w2] -> Differential equation of y_w2/21(psi_w2)
  [K_gy] -> Differential equation of y_w2/22(K_gy)
  [y_a2] -> Differential equation of y_w2/23(y_a2)
  [theta_cl2] -> Differential equation of y_w2/24(theta_cl2)
  [m_w] -> Differential equation of y_w3/1(m_w)
  [k_py] -> Differential equation of y_w3/2(k_py)
  [y_t2] -> Differential equation of y_w3/3(y_t2)
  [b] -> Differential equation of y_w3/4(b)
  [psi_t2] -> Differential equation of y_w3/5(psi_t2)
  [y_w3] -> Differential equation of y_w3/8(y_w3)
  [h_tp] -> Differential equation of y_w3/6(h_tp)
  [theta_t2] -> Differential equation of y_w3/7(theta_t2)
  [c_py] -> Differential equation of y_w3/9(c_py)
  [y_t2_dot] -> Differential equation of y_w3/10(y_t2_dot)
  [psi_t2_dot] -> Differential equation of y_w3/11(psi_t2_dot)
  [theta_t2_dot] -> Differential equation of y_w3/12(theta_t2_dot)
  [y_w3_dot] -> Differential equation of y_w3/13(y_w3_dot)
  [f_22] -> Differential equation of y_w3/14(f_22)
  [V] -> Differential equation of y_w3/15(V)
  [sigma] -> Differential equation of y_w3/16(sigma)
  [a] -> Differential equation of y_w3/18(a)
  [y_a3_dot] -> Differential equation of y_w3/19(y_a3_dot)
  [r_0] -> Differential equation of y_w3/17(r_0)
  [theta_cl3_dot] -> Differential equation of y_w3/20(theta_cl3_dot)
  [psi_w3] -> Differential equation of y_w3/21(psi_w3)
  [K_gy] -> Differential equation of y_w3/22(K_gy)
  [y_a3] -> Differential equation of y_w3/23(y_a3)
  [theta_cl3] -> Differential equation of y_w3/24(theta_cl3)
  [m_w] -> Differential equation of y_w4/1(m_w)
  [k_py] -> Differential equation of y_w4/2(k_py)
  [y_t2] -> Differential equation of y_w4/3(y_t2)
  [b] -> Differential equation of y_w4/4(b)
  [psi_t2] -> Differential equation of y_w4/5(psi_t2)
  [h_tp] -> Differential equation of y_w4/6(h_tp)
  [theta_t2] -> Differential equation of y_w4/7(theta_t2)
  [y_w4] -> Differential equation of y_w4/8(y_w4)
  [c_py] -> Differential equation of y_w4/9(c_py)
  [y_t2_dot] -> Differential equation of y_w4/10(y_t2_dot)
  [psi_t2_dot] -> Differential equation of y_w4/11(psi_t2_dot)
  [theta_t2_dot] -> Differential equation of y_w4/12(theta_t2_dot)
  [y_w4_dot] -> Differential equation of y_w4/13(y_w4_dot)
  [f_22] -> Differential equation of y_w4/14(f_22)
  [V] -> Differential equation of y_w4/15(V)
  [sigma] -> Differential equation of y_w4/16(sigma)
  [r_0] -> Differential equation of y_w4/17(r_0)
  [a] -> Differential equation of y_w4/18(a)
  [y_a4_dot] -> Differential equation of y_w4/19(y_a4_dot)
  [theta_cl4_dot] -> Differential equation of y_w4/20(theta_cl4_dot)
  [psi_w4] -> Differential equation of y_w4/21(psi_w4)
  [y_a4] -> Differential equation of y_w4/23(y_a4)
  [K_gy] -> Differential equation of y_w4/22(K_gy)
  [theta_cl4] -> Differential equation of y_w4/24(theta_cl4)
  [J_cx] -> Differential equation of theta_c/1(J_cx)
  [K_sy] -> Differential equation of theta_c/2(k_sy)
  [h_cs] -> Differential equation of theta_c/4(h_cs)
  [y_t1] -> Differential equation of theta_c/6(y_t1)
  [y_t2] -> Differential equation of theta_c/7(y_t2)
  [h_ts] -> Differential equation of theta_c/8(h_ts)
  [theta_t1] -> Differential equation of theta_c/9(theta_t1)
  [theta_t2] -> Differential equation of theta_c/10(theta_t2)
  [C_sy] -> Differential equation of theta_c/11(c_sy)
  [y_t1_dot] -> Differential equation of theta_c/14(y_t1_dot)
  [y_t2_dot] -> Differential equation of theta_c/15(y_t2_dot)
  [theta_t1_dot] -> Differential equation of theta_c/16(theta_t1_dot)
  [theta_t2_dot] -> Differential equation of theta_c/17(theta_t2_dot)
  [k_sz] -> Differential equation of theta_c/18(k_sz)
  [d_s] -> Differential equation of theta_c/19(d_s)
  [c_sz] -> Differential equation of theta_c/20(c_sz)
  [l] -> Differential equation of y_t1/4(l)
  [y_c] -> Differential equation of y_t1/3(y_c)
  [K_sy] -> Differential equation of y_t1/2(k_sy)
  [m_t] -> Differential equation of y_t1/1(m_t)
  [h_cs] -> Differential equation of y_t1/6(h_cs)
  [theta_c] -> Differential equation of y_t1/7(theta_c)
  [y_t1] -> Differential equation of y_t1/8(y_t1)
  [h_ts] -> Differential equation of y_t1/9(h_ts)
  [theta_t1] -> Differential equation of y_t1/10(theta_t1)
  [C_sy] -> Differential equation of y_t1/11(c_sy)
  [y_c_dot] -> Differential equation of y_t1/12(y_c_dot)
  [psi_c_dot] -> Differential equation of y_t1/13(psi_c_dot)
  [theta_c_dot] -> Differential equation of y_t1/14(theta_c_dot)
  [y_t1_dot] -> Differential equation of y_t1/15(y_t1_dot)
  [theta_t1_dot] -> Differential equation of y_t1/16(theta_t1_dot)
  [k_py] -> Differential equation of y_t1/17(k_py)
  [h_tp] -> Differential equation of y_t1/18(h_tp)
  [y_w1] -> Differential equation of y_t1/19(y_w1)
  [y_w2] -> Differential equation of y_t1/20(y_w2)
  [c_py] -> Differential equation of y_t1/21(c_py)
  [y_w1_dot] -> Differential equation of y_t1/22(y_w1_dot)
  [y_w2_dot] -> Differential equation of y_t1/23(y_w2_dot)
  [f_1] -> Differential equation of y_t1/24(f_1)
  [m_t] -> Differential equation of y_t2/1(m_t)
  [K_sy] -> Differential equation of y_t2/2(k_sy)
  [y_c] -> Differential equation of y_t2/3(y_c)
  [l] -> Differential equation of y_t2/4(l)
  [psi_c] -> Differential equation of y_t2/5(psi_c)
  [h_cs] -> Differential equation of y_t2/6(h_cs)
  [theta_c] -> Differential equation of y_t2/7(theta_c)
  [y_t2] -> Differential equation of y_t2/8(y_t2)
  [h_ts] -> Differential equation of y_t2/9(h_ts)
  [theta_t2] -> Differential equation of y_t2/10(theta_t2)
  [C_sy] -> Differential equation of y_t2/11(c_sy)
  [y_c_dot] -> Differential equation of y_t2/12(y_c_dot)
  [psi_c_dot] -> Differential equation of y_t2/13(psi_c_dot)
  [theta_c_dot] -> Differential equation of y_t2/14(theta_c_dot)
  [y_t2_dot] -> Differential equation of y_t2/15(y_t2_dot)
  [theta_t2_dot] -> Differential equation of y_t2/16(theta_t2_dot)
  [k_py] -> Differential equation of y_t2/17(k_py)
  [h_tp] -> Differential equation of y_t2/18(h_tp)
  [y_w3] -> Differential equation of y_t2/19(y_w3)
  [y_w4] -> Differential equation of y_t2/20(y_w4)
  [c_py] -> Differential equation of y_t2/21(c_py)
  [y_w3_dot] -> Differential equation of y_t2/22(y_w3_dot)
  [y_w4_dot] -> Differential equation of y_t2/23(y_w4_dot)
  [f_2] -> Differential equation of y_t2/24(f_2)
  [J_tz] -> Differential equation of psi_t1/1(J_tz)
  [k_sx] -> Differential equation of psi_t1/2(k_sx)
  [psi_c] -> Differential equation of psi_t1/3(psi_c)
  [psi_t1] -> Differential equation of psi_t1/4(psi_t1)
  [d_s] -> Differential equation of psi_t1/5(d_s)
  [c_sx] -> Differential equation of psi_t1/6(c_sx)
  [psi_c_dot] -> Differential equation of psi_t1/7(psi_c_dot)
  [psi_t1_dot] -> Differential equation of psi_t1/8(psi_t1_dot)
  [k_px] -> Differential equation of psi_t1/9(k_px)
  [psi_w1] -> Differential equation of psi_t1/10(psi_w1)
  [psi_w2] -> Differential equation of psi_t1/11(psi_w2)
  [d_p] -> Differential equation of psi_t1/12(d_p)
  [c_px] -> Differential equation of psi_t1/13(c_px)
  [psi_w1_dot] -> Differential equation of psi_t1/14(psi_w1_dot)
  [psi_w2_dot] -> Differential equation of psi_t1/15(psi_w2_dot)
  [k_py] -> Differential equation of psi_t1/16(k_py)
  [b] -> Differential equation of psi_t1/17(b)
  [y_w1] -> Differential equation of psi_t1/18(y_w1)
  [y_w2] -> Differential equation of psi_t1/19(y_w2)
  [c_py] -> Differential equation of psi_t1/20(c_py)
  [y_w1_dot] -> Differential equation of psi_t1/21(y_w1_dot)
  [y_w2_dot] -> Differential equation of psi_t1/22(y_w2_dot)
  [J_tz] -> Differential equation of psi_t2/1(J_tz)
  [k_sx] -> Differential equation of psi_t2/2(k_sx)
  [psi_c] -> Differential equation of psi_t2/3(psi_c)
  [psi_t2] -> Differential equation of psi_t2/4(psi_t2)
  [d_s] -> Differential equation of psi_t2/5(d_s)
  [c_sx] -> Differential equation of psi_t2/6(c_sx)
  [psi_c_dot] -> Differential equation of psi_t2/7(psi_c_dot)
  [psi_t2_dot] -> Differential equation of psi_t2/8(psi_t2_dot)
  [k_px] -> Differential equation of psi_t2/9(k_px)
  [psi_w3] -> Differential equation of psi_t2/10(psi_w3)
  [psi_w4] -> Differential equation of psi_t2/11(psi_w4)
  [d_p] -> Differential equation of psi_t2/12(d_p)
  [c_px] -> Differential equation of psi_t2/13(c_px)
  [psi_w3_dot] -> Differential equation of psi_t2/14(psi_w3_dot)
  [psi_w4_dot] -> Differential equation of psi_t2/15(psi_w4_dot)
  [k_py] -> Differential equation of psi_t2/16(k_py)
  [b] -> Differential equation of psi_t2/17(b)
  [y_w3] -> Differential equation of psi_t2/18(y_w3)
  [y_w4] -> Differential equation of psi_t2/19(y_w4)
  [c_py] -> Differential equation of psi_t2/20(c_py)
  [y_w3_dot] -> Differential equation of psi_t2/21(y_w3_dot)
  [y_w4_dot] -> Differential equation of psi_t2/22(y_w4_dot)
  [J_tx] -> Differential equation of theta_t1/1(J_tx)
  [K_sy] -> Differential equation of theta_t1/2(k_sy)
  [h_ts] -> Differential equation of theta_t1/3(h_ts)
  [y_c] -> Differential equation of theta_t1/4(y_c)
  [l] -> Differential equation of theta_t1/5(l)
  [psi_c] -> Differential equation of theta_t1/6(psi_c)
  [h_cs] -> Differential equation of theta_t1/7(h_cs)
  [theta_c] -> Differential equation of theta_t1/8(theta_c)
  [y_t1] -> Differential equation of theta_t1/9(y_t1)
  [theta_t1] -> Differential equation of theta_t1/10(theta_t1)
  [C_sy] -> Differential equation of theta_t1/11(c_sy)
  [y_c_dot] -> Differential equation of theta_t1/12(y_c_dot)
  [psi_c_dot] -> Differential equation of theta_t1/13(psi_c_dot)
  [theta_c_dot] -> Differential equation of theta_t1/14(theta_c_dot)
  [y_t1_dot] -> Differential equation of theta_t1/15(y_t1_dot)
  [theta_t1_dot] -> Differential equation of theta_t1/16(theta_t1_dot)
  [k_sz] -> Differential equation of theta_t1/17(k_sz)
  [d_s] -> Differential equation of theta_t1/18(d_s)
  [c_sz] -> Differential equation of theta_t1/19(c_sz)
  [k_py] -> Differential equation of theta_t1/20(k_py)
  [h_tp] -> Differential equation of theta_t1/21(h_tp)
  [y_w1] -> Differential equation of theta_t1/22(y_w1)
  [y_w2] -> Differential equation of theta_t1/23(y_w2)
  [c_py] -> Differential equation of theta_t1/24(c_py)
  [y_w1_dot] -> Differential equation of theta_t1/25(y_w1_dot)
  [y_w2_dot] -> Differential equation of theta_t1/26(y_w2_dot)
  [k_pz] -> Differential equation of theta_t1/27(k_pz)
  [d_p] -> Differential equation of theta_t1/28(d_p)
  [c_pz] -> Differential equation of theta_t1/29(c_pz)
  [f_1] -> Differential equation of theta_t1/30(f_1)
  [J_tx] -> Differential equation of theta_t2/1(J_tx)
  [K_sy] -> Differential equation of theta_t2/2(k_sy)
  [h_ts] -> Differential equation of theta_t2/3(h_ts)
  [y_c] -> Differential equation of theta_t2/4(y_c)
  [l] -> Differential equation of theta_t2/5(l)
  [psi_c] -> Differential equation of theta_t2/6(psi_c)
  [h_cs] -> Differential equation of theta_t2/7(h_cs)
  [theta_c] -> Differential equation of theta_t2/8(theta_c)
  [y_t2] -> Differential equation of theta_t2/9(y_t2)
  [theta_t2] -> Differential equation of theta_t2/10(theta_t2)
  [C_sy] -> Differential equation of theta_t2/11(c_sy)
  [y_c_dot] -> Differential equation of theta_t2/12(y_c_dot)
  [psi_c_dot] -> Differential equation of theta_t2/13(psi_c_dot)
  [theta_c_dot] -> Differential equation of theta_t2/14(theta_c_dot)
  [y_t2_dot] -> Differential equation of theta_t2/15(y_t2_dot)
  [theta_t2_dot] -> Differential equation of theta_t2/16(theta_t2_dot)
  [k_sz] -> Differential equation of theta_t2/17(k_sz)
  [d_s] -> Differential equation of theta_t2/18(d_s)
  [c_sz] -> Differential equation of theta_t2/19(c_sz)
  [k_py] -> Differential equation of theta_t2/20(k_py)
  [h_tp] -> Differential equation of theta_t2/21(h_tp)
  [y_w3] -> Differential equation of theta_t2/22(y_w3)
  [y_w4] -> Differential equation of theta_t2/23(y_w4)
  [c_py] -> Differential equation of theta_t2/24(c_py)
  [y_w3_dot] -> Differential equation of theta_t2/25(y_w3_dot)
  [y_w4_dot] -> Differential equation of theta_t2/26(y_w4_dot)
  [k_pz] -> Differential equation of theta_t2/27(k_pz)
  [d_p] -> Differential equation of theta_t2/28(d_p)
  [c_pz] -> Differential equation of theta_t2/29(c_pz)
  [f_2] -> Differential equation of theta_t2/30(f_2)
  [a] -> Differential equation of psi_w4/16(a)
  [a] -> "Differential equation of psi_w1 "/16(a)
  [r_0] -> "Differential equation of psi_w1 "/17(r_0)
  [r_0] -> Differential equation of psi_w2/17(r_0)
  [a] -> Differential equation of psi_w2/16(a)
  [r_0] -> Differential equation of psi_w3/17(r_0)
  [a] -> Differential equation of psi_w3/16(a)
  [r_0] -> Differential equation of psi_w4/17(r_0)
  Manual Switch34/1 -> Add49/2, To Workspace37/1, To Workspace39/1, To Workspace9/1, To Workspace8/1, To Workspace7/1, To Workspace6/1, To Workspace4/1  "y_actual"
  Integrator5/1 -> Manual Switch3/2
  Constant1/1 -> Manual Switch3/1, Manual Switch2/2
  Manual Switch4/1 -> [y_t2_dot]
  Constant2/1 -> Manual Switch4/2, Manual Switch5/1
  Manual Switch5/1 -> [y_t2]
  Integrator9/1 -> Manual Switch5/2
  Integrator8/1 -> Manual Switch4/1, Integrator9/1
  Manual Switch6/1 -> [psi_t2_dot]
  Constant3/1 -> Manual Switch7/1, Manual Switch6/2
  Manual Switch7/1 -> [psi_t2]
  Integrator12/1 -> Manual Switch7/2
  Integrator13/1 -> Manual Switch6/1, Integrator12/1
  Manual Switch8/1 -> [theta_t2_dot]
  Constant4/1 -> Manual Switch8/2, Manual Switch9/1
  Manual Switch9/1 -> [theta_t2]
  Integrator17/1 -> Manual Switch9/2
  Integrator16/1 -> Manual Switch8/1, Integrator17/1
  Manual Switch10/1 -> [psi_c_dot]
  Constant5/1 -> Manual Switch11/1, Manual Switch10/2
  Manual Switch11/1 -> [psi_c]
  Integrator3/1 -> Manual Switch11/2
  Integrator2/1 -> Manual Switch10/1, Integrator3/1
  Manual Switch12/1 -> [y_t1_dot]
  Constant6/1 -> Manual Switch13/1, Manual Switch12/2
  Manual Switch13/1 -> [y_t1]
  Integrator7/1 -> Manual Switch13/2
  Integrator6/1 -> Manual Switch12/1, Integrator7/1
  Manual Switch14/1 -> [psi_t1_dot]
  Constant7/1 -> Manual Switch14/2, Manual Switch15/1
  Manual Switch15/1 -> [psi_t1]
  Integrator11/1 -> Manual Switch15/2
  Integrator10/1 -> Manual Switch14/1, Integrator11/1
  Manual Switch16/1 -> [theta_t1_dot]
  Constant8/1 -> Manual Switch17/1, Manual Switch16/2
  Manual Switch17/1 -> [theta_t1]
  Integrator15/1 -> Manual Switch17/2
  Integrator14/1 -> Manual Switch16/1, Integrator15/1
  Manual Switch18/1 -> [y_w1_dot]
  Constant9/1 -> Manual Switch19/1, Manual Switch18/2
  Manual Switch19/1 -> [y_w1]
  Integrator19/1 -> Manual Switch19/2
  Integrator18/1 -> Manual Switch18/1, Integrator19/1
  Manual Switch20/1 -> [y_w2_dot]
  Constant10/1 -> Manual Switch21/1, Manual Switch20/2
  Manual Switch21/1 -> [y_w2]
  Integrator21/1 -> Manual Switch21/2
  Integrator20/1 -> Manual Switch20/1, Integrator21/1
  Manual Switch22/1 -> [y_w3_dot]
  Constant11/1 -> Manual Switch23/1, Manual Switch22/2
  Manual Switch23/1 -> [y_w3]
  Integrator23/1 -> Manual Switch23/2
  Integrator22/1 -> Manual Switch22/1, Integrator23/1
  Manual Switch24/1 -> [y_w4_dot]
  Constant12/1 -> Manual Switch25/1, Manual Switch24/2
  Manual Switch25/1 -> [y_w4]
  Integrator24/1 -> Manual Switch25/2
  Integrator25/1 -> Manual Switch24/1, Integrator24/1
  Manual Switch26/1 -> [psi_w1_dot]
  Constant13/1 -> Manual Switch27/1, Manual Switch26/2
  Manual Switch27/1 -> [psi_w1]
  Integrator27/1 -> Manual Switch27/2
  Integrator26/1 -> Manual Switch26/1, Integrator27/1
  Manual Switch28/1 -> [psi_w2_dot]
  Constant14/1 -> Manual Switch28/2, Manual Switch29/1
  Manual Switch29/1 -> [psi_w2]
  Integrator29/1 -> Manual Switch29/2
  Integrator28/1 -> Manual Switch28/1, Integrator29/1
  Manual Switch30/1 -> [psi_w3_dot]
  Constant15/1 -> Manual Switch31/1, Manual Switch30/2
  Manual Switch31/1 -> [psi_w3]
  Integrator31/1 -> Manual Switch31/2
  Integrator30/1 -> Manual Switch30/1, Integrator31/1
  Manual Switch32/1 -> [psi_w4_dot]
  Constant16/1 -> Manual Switch33/1, Manual Switch32/2
  Manual Switch33/1 -> [psi_w4]
  Integrator33/1 -> Manual Switch33/2
  Integrator32/1 -> Manual Switch32/1, Integrator33/1
  Constant17/1 -> Manual Switch34/1, Manual Switch1/2
  Integrator1/1 -> Manual Switch34/2
  Integrator/1 -> Manual Switch1/1, Integrator1/1
  [y_c] -> y_c/1
  From435/1 -> Goto17/1
  Subsystem3/1(Out1) -> Goto20/1
  From429/1 -> Subsystem3/1(In1)
  From480/1 -> Subsystem3/2(In2)
  Constant40/1 -> Subsystem3/3(In3)
  From418/1 -> Subsystem7/1(In1)
  From419/1 -> Subsystem7/4(In4)
  From430/1 -> Subsystem7/6(In6)
  From474/1 -> Subsystem7/7(In7)
  From475/1 -> Subsystem7/8(In8)
  From476/1 -> Subsystem7/9(In9)
  From420/1 -> Subsystem7/10(In10)
  Constant21/1 -> Subsystem7/11(In11)
  From415/1 -> Subsystem8/1(In1)
  From425/1 -> Subsystem8/2(In2)
  From426/1 -> Subsystem8/3(In3)
  From416/1 -> Subsystem8/4(In4)
  From423/1 -> Subsystem8/5(In5)
  From427/1 -> Subsystem8/6(In6)
  From449/1 -> Subsystem8/7(In7)
  From457/1 -> Subsystem8/8(In8)
  From466/1 -> Subsystem8/9(In9)
  Constant19/1 -> Subsystem8/11(In11)
  From455/1 -> Subsystem9/1(In1)
  Subsystem9/1(Out1) -> Goto39/1
  From437/1 -> Subsystem10/1(In1)
  Subsystem10/1(Out1) -> Goto42/1
  From436/1 -> Subsystem11/1(In1)
  From472/1 -> Subsystem11/2(In2)
  Subsystem11/1(Out1) -> Goto51/1
  From428/1 -> Subsystem7/3(In3)
  From432/1 -> Subsystem7/2(In2)
  From431/1 -> Subsystem7/5(In5)
  Gain1/1 -> [y_a4_dot], [y_a3_dot], [y_a2_dot], [y_a1_dot], Scope2/1
  Gain/1 -> Scope4/1, [theta_cl4_dot], [theta_cl3_dot], [theta_cl2_dot], [theta_cl1_dot]
  Manual Switch35/1 -> Goto48/1
  Subsystem7/1(Out1) -> Manual Switch35/1
  1/1 -> Manual Switch35/2
  Manual Switch/1 -> Goto45/1
  Subsystem8/1(Out1) -> Manual Switch/1
  0/1 -> Manual Switch/2
  4A_ap/pi/1 -> Product24/2
  15/1 -> Add/2
  Add/1 -> Product24/1
  35/1 -> Add/3
  3/1 -> Add/1
  Product24/1 -> Scope/1, To Workspace3/1  "ya"
  (3)/1 -> Add1/1
  99/1 -> Add1/3
  Add1/1 -> Product1/1
  4A_vp/b*pi/1 -> Product1/2
  (35)/1 -> Add1/2
  Product1/1 -> To Workspace18/1, Scope/2  "θcl"
  disturbance and noise/5(gaussian_disturbance) -> Gain2/1, Scope3/1, Gain/1, Gain1/1
  From417/1 -> Subsystem8/10(In10)
  Clock2/1 -> F_wind/1(t)
  [V] -> F_wind/2(v_train)
  F_wind/1(F_side) -> Gain3/1, Scope7/1
  F_wind/2(M_roll) -> Gain4/1
  Differential equation of y_c/1(y_c_ddot) -> Integrator/1, To Workspace16/1, To Workspace14/1, To Workspace13/1, To Workspace12/1, To Workspace11/1, To Workspace38/1, To Workspace36/1, [y_c_ddot]  "ycdd"
  F_wind/3(w_c) -> Scope8/1
  [y_c_dot] -> Differential equation of y_c/12(y_c_dot)
  Manual Switch1/1 -> To Workspace22/1, To Workspace17/1, To Workspace43/1, To Workspace10/1, To Workspace21/1, To Workspace23/1, Add24/1
  Add24/1 -> [y_c_dot]
  disturbance and noise/7(actual_sensor_noise_acc_highsamplingfreq) -> [noise]
  [noise_v] -> Add24/2  "Noise_v"
  Gain2/1 -> [noise_phi]
  Add9/1 -> To Workspace42/1, To Workspace31/1, To Workspace2/1, To Workspace28/1, To Workspace29/1, To Workspace30/1, [theta_c_dot]
  Manual Switch2/1 -> Add9/1
  [noise_w] -> Add9/2  "noisy_w"
  [f_1] -> Differential equation of theta_c/21(f_1)
  [f_2] -> Differential equation of theta_c/22(f_2)
  Manual Switch3/1 -> To Workspace24/1, To Workspace25/1, To Workspace27/1, To Workspace26/1, To Workspace41/1, To Workspace5/1, Add14/2  "phic_actual"
  Add14/1 -> [theta_c]
  Gain3/1 -> To Workspace1/1, [F_wind]
  Gain4/1 -> Scope25/1, [M_wind]
  Differential equation of theta_c/2(y1) -> Scope40/1  "状态1"
  Differential equation of theta_c/3(y2) -> Scope40/2  "状态2"
  Differential equation of theta_c/4(y3) -> Scope40/3  "垂直"
  Differential equation of y_c/2(y1) -> Scope49/1  "状态"
  Differential equation of y_c/3(y2) -> Scope49/2  "扰动"
  Differential equation of y_c/4(y3) -> Scope49/3  "输入"
  Differential equation of theta_c/5(y4) -> Scope40/4  "控制输入"
  Differential equation of theta_c/6(y5) -> Scope40/5  "wind"
  Differential equation of y_c/5(y4) -> Scope49/4
  Differential equation of y_c/6(y5) -> Scope49/5  "f_wind"
  Differential equation of theta_c/7(y6) -> Scope40/6
  Differential equation of y_c/7(y6) -> Scope49/6
  [F_wind] -> Differential equation of theta_c/23(F_wind)
  [F_wind] -> Differential equation of y_c/20(F_wind)
  Differential equation of theta_c/1(theta_c_ddot) -> Integrator4/1, To Workspace40/1, To Workspace35/1, To Workspace15/1, To Workspace32/1, To Workspace33/1, To Workspace34/1
  Add25/1 -> [K_sy]
  Clock17/1 -> MATLAB Function16/1(t)
  MATLAB Function16/1(y) -> Add25/2
  k_sy/1 -> Add25/1
  Add10/1 -> [C_sy]
  Clock10/1 -> MATLAB Function8/1(t)
  MATLAB Function8/1(y) -> Add10/2
  "c_sy "/1 -> Add10/1
  Clock9/1 -> MATLAB Function9/1(t)
  Add15/1 -> [M_c]
  m_c/1 -> Add15/1
  MATLAB Function9/1(y) -> Add15/2
  Gain5/1 -> Add17/1
  Integrator35/1 -> Add21/1, Gain8/1
  Band-Limited White Noise5/1 -> Add19/2, Scope32/1
  Add20/1 -> Goto155/1, Integrator35/1
  Gain7/1 -> Add18/2
  Add21/1 -> To Workspace20/1, [noise_w], Subtract1/1  "noise_w"
  Atan2/1 -> Gain5/1, Subtract/2
  Integrator38/1 -> To Workspace19/1, [noise_v]  "noise_v"
  Add16/1 -> Subtract1/2
  Add18/1 -> Integrator36/1
  Constant34/1 -> Atan2/2
  Gain9/1 -> Integrator34/1
  Integrator36/1 -> Scope31/1, Add19/1, Gain7/1
  Band-Limited White Noise4/1 -> Add18/1
  Add19/1 -> Goto154/1, Integrator38/1, Atan2/1
  Gain10/1 -> Add17/2
  Integrator37/1 -> Gain10/1
  Band-Limited White Noise7/1 -> Add21/2
  Gain8/1 -> Add20/2
  Gain6/1 -> Add16/1
  Add17/1 -> To Workspace44/1, [noise_sheta], Subtract/1, Scope30/1
  Subtract/1 -> Gain9/1, Gain6/1
  Band-Limited White Noise6/1 -> Add20/1
  Integrator34/1 -> Add16/2
  Subtract1/1 -> Integrator37/1
  sigma/1 -> [sigma]
  "c_sz "/1 -> [c_sz]
  J_cz/1 -> [J_cz]
  f_22/1 -> [f_22]
  h_cs/1 -> [h_cs]
  c_px/1 -> [c_px]
  V/1 -> [V]
  "h_ts "/1 -> [h_ts]
  " "/1 -> [Lambda_v]
  Constant30/1 -> [T1]
  k24/1 -> [k24]
  k_sx/1 -> [k_sx]
  "J_tx "/1 -> [J_tx]
  l_t/1 -> [b]
  b/1 -> [a]
  M_t/1 -> [m_t]
  k_px/1 -> [k_px]
  k23/1 -> [k23]
  Lambda_a/1 -> [Lambda_a]
  J_cx/1 -> [J_cx]
  lambda_e/1 -> [lambda_e]
  Omega_c/1 -> [Omega_c]
  Constant33/1 -> [T2]
  k12/1 -> [k12]
  k14/1 -> [k14]
  k13/1 -> [k13]
  k2/1 -> [k22]
  J_wz/1 -> [J_wz]
  Tnn/1 -> [Tnn]
  Tff/1 -> [Tff]
  "k_py "/1 -> [k_py]
  kp/1 -> [kp]
  l_c/1 -> [l]
  d_p/1 -> [d_p]
  Omega_r/1 -> [Omega_r]
  r_0/1 -> [r_0]
  k_sz/1 -> [k_sz]
  d_s/1 -> [d_s]
  K_gpsi/1 -> [K_gpsi]
  "c_pz "/1 -> [c_pz]
  "J_tz "/1 -> [J_tz]
  k1/1 -> [k21]
  c_py/1 -> [c_py]
  k11/1 -> [k11]
  k_pz/1 -> [k_pz]
  c_sx/1 -> [c_sx]
  K_gy/1 -> [K_gy]
  kd/1 -> [kd]
  f_11/1 -> [f_11]
  h_tw/1 -> [h_tp]
  M_w/1 -> [m_w]
  Omega_s/1 -> [Omega_s]
  Band-Limited White Noise/1 -> Transfer Fcn2/1, Transfer Fcn3/1
  Transfer Fcn2/1 -> [lateral_alignment], Scope1/1  "L"
  Transfer Fcn3/1 -> [cross_level], Scope1/2  "C"
  [lateral_alignment] -> [y_a1], [y_a4], [y_a3], [y_a2]
  [cross_level] -> Gain21/1
  Gain21/1 -> [theta_cl4], [theta_cl3], [theta_cl2], [theta_cl1]
  Differential equation of psi_c/1(psi_c_ddot) -> Integrator2/1
  From836/1 -> Product57/2
  Product59/1 -> Add47/3
  Gain24/1 -> Goto173/1
  From833/1 -> Product59/2
  Product51/1 -> Add43/1
  From812/1 -> Add39/1
  Product58/1 -> Add48/2
  Gain23/1 -> Goto166/1
  From829/1 -> Add45/1
  Add39/1 -> MATLAB Function6/1(sigma_t)
  From814/1 -> Add38/1
  Product56/1 -> Add47/1
  MATLAB Function10/1(y) -> Add47/4
  k5/1 -> Product56/1
  From826/1 -> Product53/2
  Add45/1 -> Goto167/1
  Constant57/1 -> Product49/2
  Add41/1 -> Goto164/1
  From832/1 -> Add46/2
  From830/1 -> Add45/2
  MATLAB Function7/1(y) -> Add43/4
  From828/1 -> MATLAB Function7/1(i)
  Add48/1 -> Product59/1
  Product54/1 -> Add43/3
  From819/1 -> Add41/1
  k1'2/1 -> Product53/1
  Product52/1 -> Add44/1
  Product50/1 -> Add43/2
  From813/1 -> Add8/1
  From815/1 -> Product47/1
  Product53/1 -> Add44/2
  From825/1 -> Product52/2
  k4/1 -> Product51/1
  From821/1 -> Add42/1
  c4/1 -> Product50/2
  Add42/1 -> Goto165/1
  From824/1 -> Product51/2
  From820/1 -> Add41/2
  Product49/1 -> Add40/2
  Add43/1 -> Gain23/1
  From817/1 -> Product49/1
  From822/1 -> Add42/2
  From804/1 -> Product48/1
  Product46/1 -> Add8/2
  Constant44/1 -> Product46/2
  From816/1 -> Add40/1
  Product47/1 -> Add38/2
  MATLAB Function5/1(uc) -> Integrator41/1
  c6/1 -> Product55/2
  Integrator41/1 -> Goto162/1  "ic"
  MATLAB Function6/1(ut) -> Integrator42/1
  Add8/1 -> MATLAB Function5/1(sigma_c)
  From839/1 -> MATLAB Function10/1(i)
  c5/1 -> Product52/1
  c7/1 -> Product57/1
  From803/1 -> Product46/1
  Constant56/1 -> Product48/2
  Add44/1 -> Product54/1
  Add38/1 -> MATLAB Function5/2(sigma_dot_c)
  Add40/1 -> MATLAB Function6/2(sigma_dot_t)
  From834/1 -> Product55/1
  From831/1 -> Add46/1
  Add47/1 -> Gain24/1
  From818/1 -> Product54/2
  Product55/1 -> Add47/2
  k1'3/1 -> Product58/1
  Constant45/1 -> Product47/2
  Product57/1 -> Add48/1
  From837/1 -> Product58/2
  From827/1 -> MATLAB Function7/2(x)
  Product48/1 -> Add39/2
  From835/1 -> Product56/2
  From823/1 -> Product50/1
  Add46/1 -> Goto168/1
  From838/1 -> MATLAB Function10/2(x)
  Integrator42/1 -> Goto163/1  "it"
  w_wind1/1 -> Manual Switch53/1
  w_wind4/1 -> Manual Switch53/2
  Manual Switch53/1 -> Manual Switch54/2
  w_wind/1 -> Manual Switch54/1
  Manual Switch54/1 -> F_wind/3(w_mean)
  [noise_sheta] -> Add14/1
  Tnn2/1 -> ?
  Tff2/1 -> ?
  From869/1 -> UDE1/3(phic)
  Gain26/1 -> Scope10/1, Goto176/1
  UDE1/1(F_1) -> Manual Switch56/1
  From878/1 -> UDE1/9(F1)
  23/1 -> Manual Switch56/2
  From870/1 -> UDE1/4(dphic)
  From874/1 -> UDE1/5(k11)
  From863/1 -> UDE1/2(dyc)
  From861/1 -> UDE1/1(yc)
  Manual Switch56/1 -> Gain26/1
  From875/1 -> UDE1/6(k12)
  From876/1 -> UDE1/7(k13)
  From879/1 -> UDE1/10(F2)
  From877/1 -> UDE1/8(k14)
  From868/1 -> UDE2/7(k13)
  From871/1 -> UDE2/8(k14)
  From873/1 -> UDE2/10(F2)
  Manual Switch57/1 -> Gain27/1
  From865/1 -> UDE2/6(k12)
  From864/1 -> UDE2/5(k11)
  From862/1 -> UDE2/4(dphic)
  From872/1 -> UDE2/9(F1)
  24/1 -> Manual Switch57/2
  From855/1 -> UDE2/2(dyc)
  UDE2/1(F_1) -> Manual Switch57/1
  From856/1 -> UDE2/3(phic)
  From854/1 -> UDE2/1(yc)
  Gain27/1 -> Scope33/1, Goto179/1
  [niose_yc] -> Add49/1
  Add49/1 -> [y_c]
  UDE+MEE4（新）10/1(F_1) -> Manual Switch58/1
  Gain28/1 -> Scope14/1, Goto181/1
  From891/1 -> UDE+MEE4（新）10/4(dphic)
  From895/1 -> UDE+MEE4（新）10/5(k11)
  25/1 -> Manual Switch58/2
  From897/1 -> UDE+MEE4（新）10/7(k13)
  From890/1 -> UDE+MEE4（新）10/3(phic)
  From898/1 -> UDE+MEE4（新）10/8(k14)
  From886/1 -> UDE+MEE4（新）10/2(dyc)
  From884/1 -> UDE+MEE4（新）10/1(yc)
  From900/1 -> UDE+MEE4（新）10/10(F2)
  Manual Switch58/1 -> Gain28/1
  From896/1 -> UDE+MEE4（新）10/6(k12)
  From899/1 -> UDE+MEE4（新）10/9(F1)
  From893/1 -> UDE+MEE4（新）8/9(F1)
  From894/1 -> UDE+MEE4（新）8/10(F2)
  From881/1 -> UDE+MEE4（新）8/1(yc)
  From882/1 -> UDE+MEE4（新）8/2(dyc)
  From888/1 -> UDE+MEE4（新）8/6(k12)
  Manual Switch59/1 -> Gain29/1
  From892/1 -> UDE+MEE4（新）8/8(k14)
  From889/1 -> UDE+MEE4（新）8/7(k13)
  From887/1 -> UDE+MEE4（新）8/5(k11)
  From885/1 -> UDE+MEE4（新）8/4(dphic)
  26/1 -> Manual Switch59/2
  UDE+MEE4（新）8/1(F_1) -> Manual Switch59/1
  From883/1 -> UDE+MEE4（新）8/3(phic)
  Gain29/1 -> Scope34/1, Goto182/1
  Band-Limited White Noise1/1 -> To Workspace46/1, [niose_yc], Scope35/1
